simulink model "PID0"  (R2020a)
settings: Solver=ode15s  StartTime=0.0  StopTime=0.4  RelTol=1e-3
values from neighbouring files (symbols this model uses):
  D = 0.0    [ModelData1.sldd]
  I = 1.0    [ModelData1.sldd]
  P = 1.0    [ModelData1.sldd]
settings Model: DataDictionary=ModelData1.sldd  Creator=tnradm  LastModifiedBy=tnradm
settings DataIOCC: SaveOutput=off  SaveTime=off

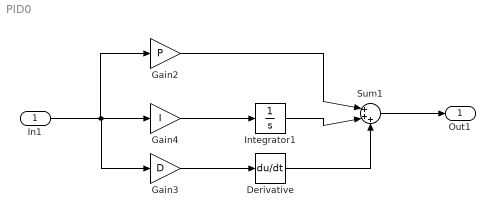
== system PID0 ==
  In1 : Inport  OutDataTypeStr=double  PortDimensions=1  SampleTime=0
  Derivative : Derivative
  Gain2 : Gain  Gain=P
  Gain3 : Gain  Gain=D
  Gain4 : Gain  Gain=I
  Integrator1 : Integrator
  Sum1 : Sum  Inputs=|+++
  Out1 : Outport  OutDataTypeStr=double  PortDimensions=1  SampleTime=0
  wires:
  In1/1 -> Gain3/1, Gain4/1, Gain2/1
  Integrator1/1 -> Sum1/2
  Derivative/1 -> Sum1/3
  Gain3/1 -> Derivative/1
  Sum1/1 -> Out1/1
  Gain2/1 -> Sum1/1
  Gain4/1 -> Integrator1/1
